simulink model "actuator_controller_inner"  (R2021b)
settings: Solver=VariableStepAuto  StartTime=0.0  StopTime=50  RelTol=1e-3
values from neighbouring files (symbols this model uses):
  K_inner_act = K_inner*0.05    [analyze_actuator_control.m]
libraries: simulink_extras x2
settings Model: Creator=austm  LastModifiedBy=austm

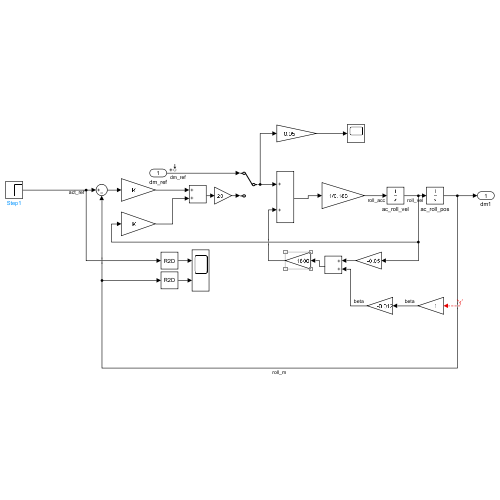
[thumbnail: Simulink's stored preview of the top-level diagram]
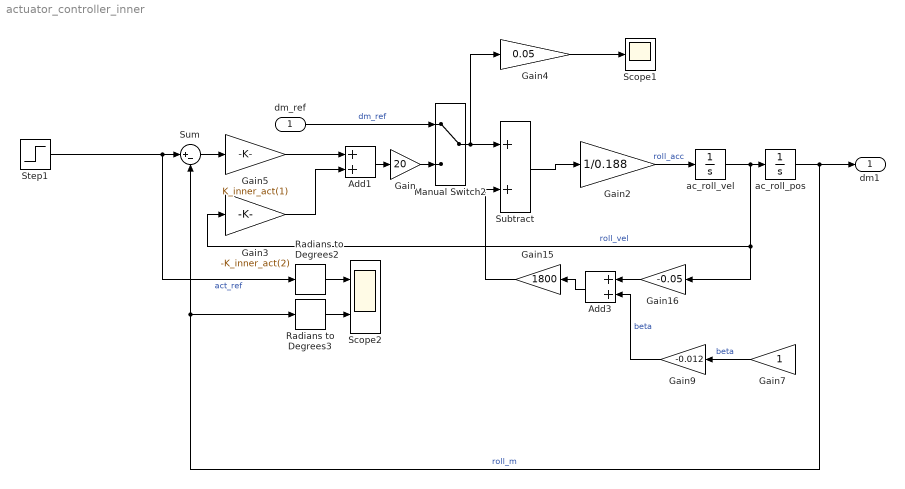
== system actuator_controller_inner ==
  dm_ref : Inport
  Add1 : Sum
  Add3 : Sum
  Gain : Gain  Gain=20
  Gain15 : Gain  Gain=1800
  Gain16 : Gain  Gain=-0.05
  Gain2 : Gain  Gain=1/0.188
  Gain3 : Gain  Gain=-K_inner_act(2)
  Gain4 : Gain  Gain=0.05
  Gain5 : Gain  Gain=K_inner_act(1)
  Gain7 : Gain
  Gain9 : Gain  Gain=-0.012
  Manual Switch2 : ManualSwitch
  Radians to Degrees2 : simulink_extras/Transformations/Radians to Degrees
  Radians to Degrees3 : simulink_extras/Transformations/Radians to Degrees
  Scope1 : Scope
  Scope2 : Scope  NumInputPorts=2
  Step1 : Step  After=0.2  SampleTime=0
  Subtract : Sum
  Sum : Sum  Inputs=|+-
  ac_roll_pos : Integrator  UpperSaturationLimit=100  LowerSaturationLimit=-100
  ac_roll_vel : Integrator  UpperSaturationLimit=100  LowerSaturationLimit=-100
  dm1 : Outport
  wires:
  ac_roll_pos/1 -> Radians to Degrees3/1, Sum/2, dm1/1  "roll_m"
  Gain2/1 -> ac_roll_vel/1  "roll_acc"
  Subtract/1 -> Gain2/1
  Manual Switch2/1 -> Gain4/1, Subtract/1
  ac_roll_vel/1 -> Gain16/1, Gain3/1, ac_roll_pos/1  "roll_vel"
  dm_ref/1 -> Manual Switch2/1  "dm_ref"
  Gain5/1 -> Add1/1
  Step1/1 -> Radians to Degrees2/1, Sum/1  "act_ref"
  Gain/1 -> Manual Switch2/2
  Gain4/1 -> Scope1/1
  Sum/1 -> Gain5/1
  Gain15/1 -> Subtract/2
  Radians to Degrees3/1 -> Scope2/2
  Radians to Degrees2/1 -> Scope2/1
  Gain16/1 -> Add3/1
  Add1/1 -> Gain/1
  Gain3/1 -> Add1/2
  Gain7/1 -> Gain9/1  "beta"
  Gain9/1 -> Add3/2  "beta"
  ? -> Gain7/1
  Add3/1 -> Gain15/1
